simulink model "simulink_discret"  (R2022b)
settings: Solver=VariableStepAuto  StartTime=0.0  StopTime=10.0  RelTol=1e-3
undefined symbols (not defined in the file): alpha_d1, beta_d1, beta_i1, beta_t1, beta_t1s, com1_max, com1_min, h1, H_1, Kp1
settings Model: Creator=Andreea  LastModifiedBy=Andreea

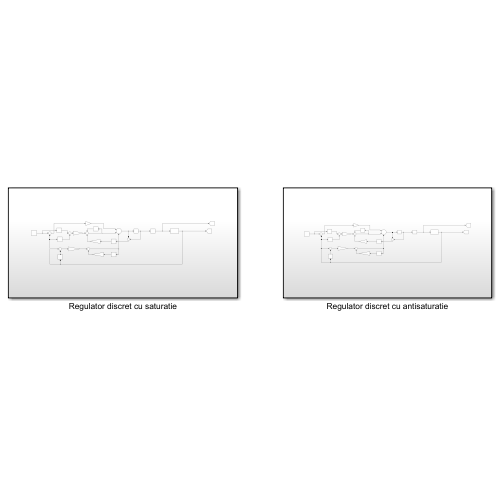
[thumbnail: Simulink's stored preview of the top-level diagram]
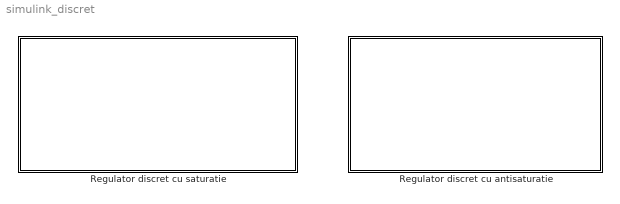
== system simulink_discret ==
  Regulator discret cu antisaturatie : Subsystem
  Regulator discret cu saturatie : Subsystem

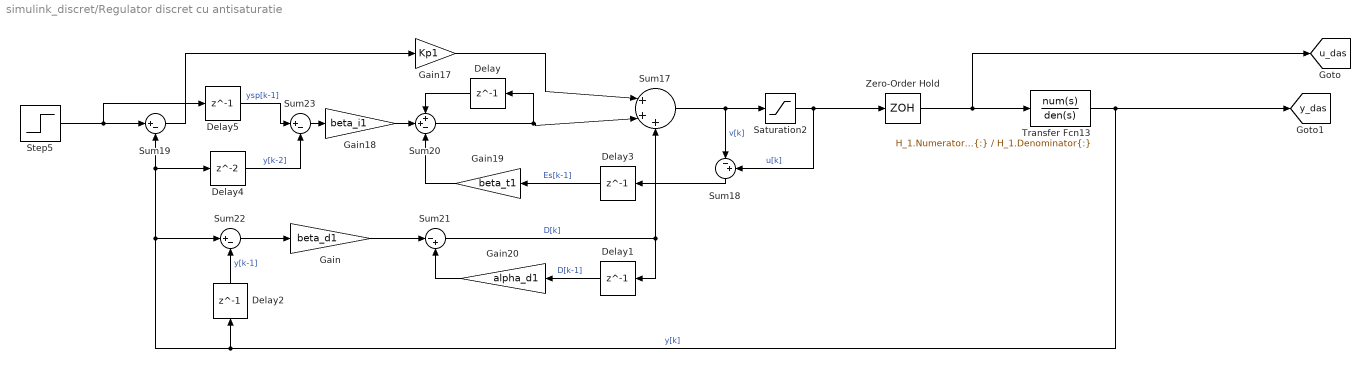
== system simulink_discret/Regulator discret cu antisaturatie ==
  Delay{,1..3,5} (5 alike) : Delay  DelayLength=1  SampleTime=h1
  Delay4 : Delay  SampleTime=h1
  Gain : Gain  Gain=beta_d1
  Gain17 : Gain  Gain=Kp1
  Gain18 : Gain  Gain=beta_i1
  Gain19 : Gain  Gain=beta_t1
  Gain20 : Gain  Gain=alpha_d1
  Saturation2 : Saturate  UpperLimit=com1_max  LowerLimit=com1_min
  Step5 : Step  Time=15  Before=1  After=0  SampleTime=0
  Sum17 : Sum  Inputs=|+++
  Sum18 : Sum  Inputs=|-+
  Sum19 : Sum  Inputs=|+-
  Sum20 : Sum  Inputs=++-
  Sum21 : Sum  Inputs=|-+
  Sum22 : Sum  Inputs=|+-
  Sum23 : Sum  Inputs=|+-
  Transfer Fcn13 : TransferFcn  Numerator=H_1.Numerator{:}  Denominator=H_1.Denominator{:}
  Zero-Order Hold : ZeroOrderHold  SampleTime=h1
  tag scope: u_das=global, y_das=global
  wires:
  Zero-Order Hold/1 -> [u_das], Transfer Fcn13/1
  Transfer Fcn13/1 -> Delay2/1, Sum22/1, Delay4/1, Sum19/2, [y_das]  "y[k]"
  Step5/1 -> Delay5/1, Sum19/1
  Delay/1 -> Sum20/1
  Gain17/1 -> Sum17/1
  Sum21/1 -> Delay1/1, Sum17/3  "D[k]"
  Sum23/1 -> Gain18/1
  Delay3/1 -> Gain19/1  "Es[k-1]"
  Sum20/1 -> Delay/1, Sum17/2
  Sum17/1 -> Saturation2/1, Sum18/1  "v[k]"
  Saturation2/1 -> Zero-Order Hold/1, Sum18/2  "u[k]"
  Delay2/1 -> Sum22/2  "y[k-1]"
  Delay1/1 -> Gain20/1  "D[k-1]"
  Delay4/1 -> Sum23/2  "y[k-2]"
  Gain18/1 -> Sum20/2
  Delay5/1 -> Sum23/1  "ysp[k-1]"
  Gain20/1 -> Sum21/2
  Sum19/1 -> Gain17/1
  Sum18/1 -> Delay3/1
  Sum22/1 -> Gain/1
  Gain19/1 -> Sum20/3
  Gain/1 -> Sum21/1

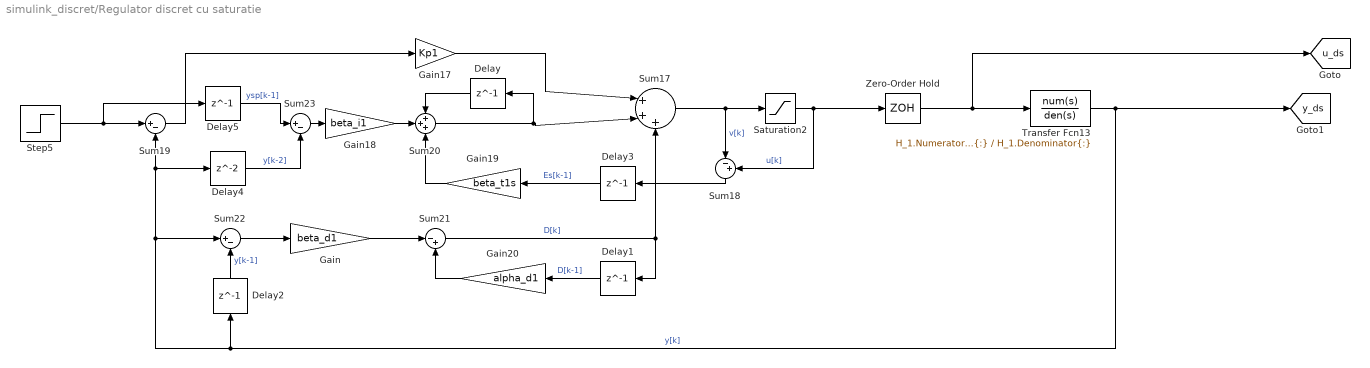
== system simulink_discret/Regulator discret cu saturatie ==
  Delay{,1..3,5} (5 alike) : Delay  DelayLength=1  SampleTime=h1
  Delay4 : Delay  SampleTime=h1
  Gain : Gain  Gain=beta_d1
  Gain17 : Gain  Gain=Kp1
  Gain18 : Gain  Gain=beta_i1
  Gain19 : Gain  Gain=beta_t1s
  Gain20 : Gain  Gain=alpha_d1
  Saturation2 : Saturate  UpperLimit=com1_max  LowerLimit=com1_min
  Step5 : Step  Time=15  Before=1  After=0  SampleTime=0
  Sum17 : Sum  Inputs=|+++
  Sum18 : Sum  Inputs=|-+
  Sum19 : Sum  Inputs=|+-
  Sum20 : Sum  Inputs=+++
  Sum21 : Sum  Inputs=|-+
  Sum22 : Sum  Inputs=|+-
  Sum23 : Sum  Inputs=|+-
  Transfer Fcn13 : TransferFcn  Numerator=H_1.Numerator{:}  Denominator=H_1.Denominator{:}
  Zero-Order Hold : ZeroOrderHold  SampleTime=h1
  tag scope: u_ds=global, y_ds=global
  wires:
  Zero-Order Hold/1 -> [u_ds], Transfer Fcn13/1
  Transfer Fcn13/1 -> Delay2/1, Delay4/1, Sum19/2, Sum22/1, [y_ds]  "y[k]"
  Step5/1 -> Delay5/1, Sum19/1
  Delay/1 -> Sum20/1
  Gain17/1 -> Sum17/1
  Sum21/1 -> Delay1/1, Sum17/3  "D[k]"
  Sum23/1 -> Gain18/1
  Delay3/1 -> Gain19/1  "Es[k-1]"
  Sum20/1 -> Delay/1, Sum17/2
  Sum17/1 -> Saturation2/1, Sum18/1  "v[k]"
  Saturation2/1 -> Zero-Order Hold/1, Sum18/2  "u[k]"
  Delay2/1 -> Sum22/2  "y[k-1]"
  Delay1/1 -> Gain20/1  "D[k-1]"
  Delay4/1 -> Sum23/2  "y[k-2]"
  Gain18/1 -> Sum20/2
  Delay5/1 -> Sum23/1  "ysp[k-1]"
  Gain20/1 -> Sum21/2
  Sum19/1 -> Gain17/1
  Sum18/1 -> Delay3/1
  Sum22/1 -> Gain/1
  Gain19/1 -> Sum20/3
  Gain/1 -> Sum21/1
